simulink model "pollaica"  (R2021a)
settings: Solver=VariableStepAuto  StartTime=0.0  StopTime=10.0  RelTol=1e-3
settings Model: Creator=Pablo Carmona  LastModifiedBy=Pablo Carmona

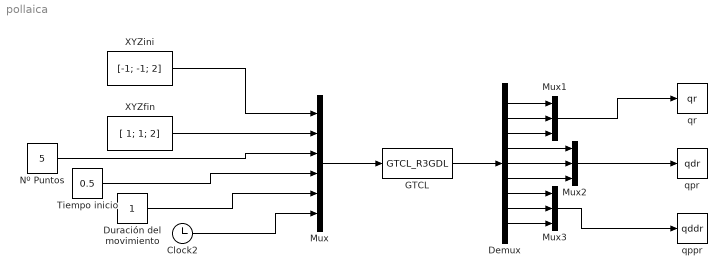
== system pollaica ==
  Clock2 : Clock
  Demux : Demux  Outputs=9
  Duración del movimiento : Constant
  GTCL : MATLABFcn  MATLABFcn=GTCL_R3GDL  OutputDimensions=9
  Mux : Mux  Inputs=6
  Mux1 : Mux  Inputs=3
  Mux2 : Mux  Inputs=3
  Mux3 : Mux  Inputs=3
  Nº Puntos : Constant  Value=5
  Tiempo inicio : Constant  Value=0.5
  XYZfin : Constant  Value=[ 1; 1; 2]
  XYZini : Constant  Value=[-1; -1; 2]
  qppr : ToWorkspace  VariableName=qddr  SampleTime=-1
  qpr : ToWorkspace  VariableName=qdr  SampleTime=-1
  qr : ToWorkspace  VariableName=qr  SampleTime=-1
  wires:
  Duración del movimiento/1 -> Mux/5
  Nº Puntos/1 -> Mux/3
  Tiempo inicio/1 -> Mux/4
  XYZini/1 -> Mux/1
  XYZfin/1 -> Mux/2
  Clock2/1 -> Mux/6
  Mux/1 -> GTCL/1
  Demux/9 -> Mux3/3
  Mux1/1 -> qr/1
  Demux/4 -> Mux2/1
  Demux/2 -> Mux1/2
  Demux/3 -> Mux1/3
  Demux/7 -> Mux3/1
  Demux/8 -> Mux3/2
  Demux/6 -> Mux2/3
  Demux/5 -> Mux2/2
  Demux/1 -> Mux1/1
  GTCL/1 -> Demux/1
  Mux2/1 -> qpr/1
  Mux3/1 -> qppr/1
